simulink model "Our_model"  (R2024b)
settings: Solver=VariableStepAuto  StartTime=0.0  StopTime=50  MaxStep=0.01  RelTol=1e-3
model workspace: external: MATLAB File Non_Linear_Model_R2024a_saveas.m (data not in the file)
libraries: slpidlib x2
settings Model: Creator=tomkl  LastModifiedBy=tomkl

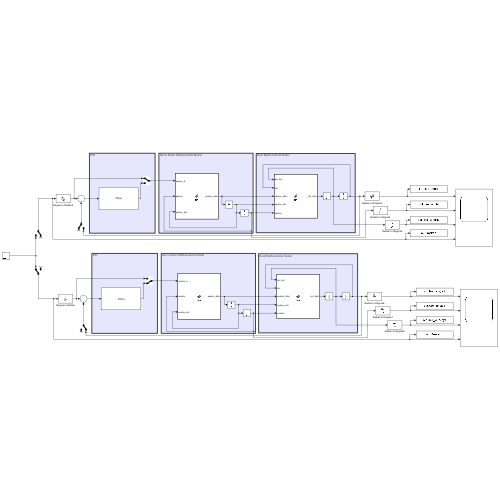
[thumbnail: Simulink's stored preview of the top-level diagram]
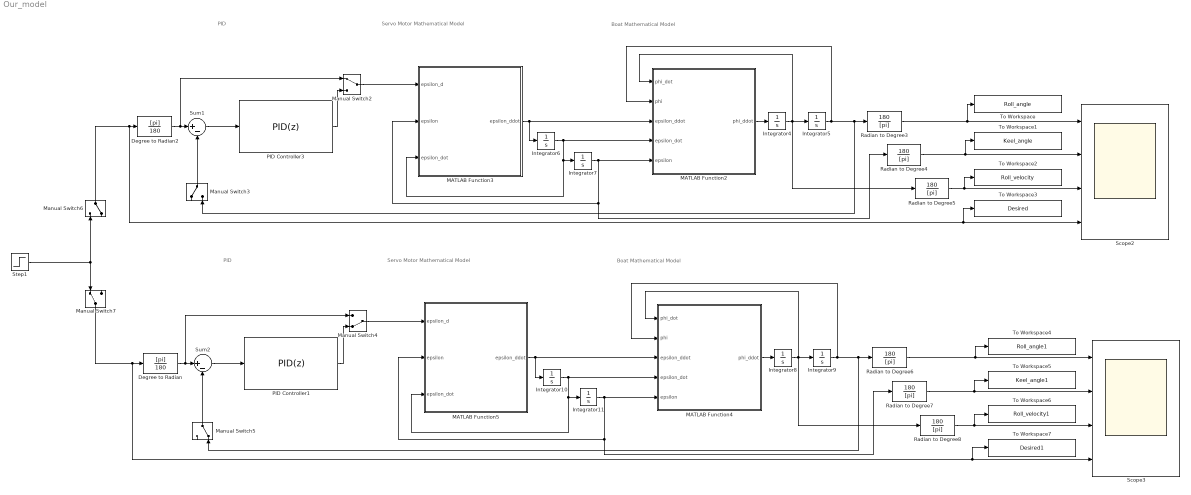
== system Our_model ==
  note: PID
  note: Boat Mathematical Model
  note: PID
  note: Servo Motor Mathematical Model
  note: Boat Mathematical Model
  note: Servo Motor Mathematical Model
  Degree to Radian : TransferFcn  Numerator=[pi]  Denominator=[180]
  Degree to Radian2 : TransferFcn  Numerator=[pi]  Denominator=[180]
  Integrator{4..11} (8 alike) : Integrator
  MATLAB Function2 : MATLAB Function  TreatAsAtomicUnit=on
  MATLAB Function3 : MATLAB Function  TreatAsAtomicUnit=on
  MATLAB Function4 : MATLAB Function  TreatAsAtomicUnit=on
  MATLAB Function5 : MATLAB Function  TreatAsAtomicUnit=on
  Manual Switch2 : ManualSwitch
  Manual Switch3 : ManualSwitch
  Manual Switch4 : ManualSwitch  CurrentSetting=0
  Manual Switch5 : ManualSwitch  CurrentSetting=0
  Manual Switch6 : ManualSwitch  CurrentSetting=0
  Manual Switch7 : ManualSwitch
  PID Controller1 : slpidlib/PID Controller  Controller=PID  Form=Parallel  TimeDomain=Discrete-time  UseExternalTs=off  SampleTime=0.01  IntegratorMethod=Forward Euler  FilterMethod=Forward Euler  ControllerParametersSource=internal  P=.8  I=0  UseKiTs=off  D=0  UseExternalDerivativeSource=off  N=1.7  UseFilter=on  TunerSelectOption=Transfer Function Based (PID Tuner App)  InitialConditionSource=internal  InitialConditionForIntegrator=0  InitialConditionForFilter=0  DifferentiatorICPrevScaledInput=0  ExternalReset=none  TrackingMode=off  Kt=1  LimitOutput=off  SatLimitsSource=internal  UpperSaturationLimit=inf  LowerSaturationLimit=-inf  LinearizeAsGain=on  AntiWindupMode=none  Kb=1  LimitIntegrator=off  UpperIntegratorSaturationLimit=inf  LowerIntegratorSaturationLimit=-inf  POutMin=[]  POutMax=[]  IOutMin=[]  IOutMax=[]  DOutMin=[]  DOutMax=[]  NOutMin=[]  NOutMax=[]  SumOutMin=[]  SumOutMax=[]  SaturationOutMin=[]  SaturationOutMax=[]  PParamMin=[]  PParamMax=[]  IParamMin=[]  IParamMax=[]  DParamMin=[]  DParamMax=[]  NParamMin=[]  NParamMax=[]  KbParamMin=[]  KbParamMax=[]  KtParamMin=[]  KtParamMax=[]  KbOutMin=[]  KbOutMax=[]  KtOutMin=[]  KtOutMax=[]  IntegratorOutMin=[]  IntegratorOutMax=[]  FilterOutMin=[]  FilterOutMax=[]  SumI1OutMin=[]  SumI1OutMax=[]  SumI2OutMin=[]  SumI2OutMax=[]  SumI3OutMin=[]  SumI3OutMax=[]  SumI4OutMin=[]  SumI4OutMax=[]  SumDOutMin=[]  SumDOutMax=[]  DifferentiatorOutMin=[]  DifferentiatorOutMax=[]  FilterDiffOutCoefMin=[]  FilterDiffOutCoefMax=[]  ReciprocalOutMin=[]  ReciprocalOutMax=[]  SumDenOutMin=[]  SumDenOutMax=[]  SumNumOutMin=[]  SumNumOutMax=[]  DivideOutMin=[]  DivideOutMax=[]  UdiffTsProdOutMin=[]  UdiffTsProdOutMax=[]  NTsProdOutMin=[]  NTsProdOutMax=[]  UintegralTsProdOutMin=[]  UintegralTsProdOutMax=[]  UngainTsProdOutMin=[]  UngainTsProdOutMax=[]  ClampingZeroOutDataTypeStr=Inherit: Inherit via back propagation  ClampingZeroOutMin=[]  ClampingZeroOutMax=[]  FilterDenConstantOutDataTypeStr=Inherit: Inherit via back propagation  FilterDenConstantOutMin=[]  FilterDenConstantOutMax=[]  PCopyOutDataTypeStr=Inherit: Inherit via back propagation  PCopyOutMin=[]  PCopyOutMax=[]  NCopyOutDataTypeStr=Inherit: Inherit via back propagation  NCopyOutMin=[]  NCopyOutMax=[]  IntegratorContinuousStateAttributes=''  IntegratorStateMustResolveToSignalObject=off  IntegratorRTWStateStorageClass=Auto  FilterContinuousStateAttributes=''  FilterStateMustResolveToSignalObject=off  FilterRTWStateStorageClass=Auto  ParallelPVariant=InternalParameters  IdealPVariant=Disabled  IVariant=InternalParameters  DVariant=InternalParameters  IntegratorVariant=Discrete  SatVariant=Disabled  AWVariant=Passthrough  PCopyVariant=Disabled  TRVariant=Disabled  FdbkBlocksVariant=Forward  IdealPFdbkVariant=Disabled  SatFdbkVariant=Disabled  DerivativeFilterVariant=ForwardEulerFilter  NVariant=InternalParameters  NCopyVariant=Disabled  FilterICVariant=InternalICsFilter  IntegratorICVariant=InternalICs  ExternalResetVariant=Disabled  TRSumVariant=Passthrough  SumFdbkVariant=Disabled  SumVariant=Sum_PID  TsampFilterVariant=InternalTs  TsampNgainVariant=Passthrough  TsampIntegralVariant=Disabled_SignalSpec  ExternalSaturationOutDataTypeStr=Inherit: Same as second input  DerivativeSourceVariant=ErrorSignal  PreIntVariant=InternalPreInt
  PID Controller3 : slpidlib/PID Controller  Controller=PID  Form=Parallel  TimeDomain=Discrete-time  UseExternalTs=off  SampleTime=0.01  IntegratorMethod=Forward Euler  FilterMethod=Forward Euler  ControllerParametersSource=internal  P=0.566467721992697  I=0.110964200934941  UseKiTs=off  D=0.339704255295508  UseExternalDerivativeSource=off  N=1.35164961739647  UseFilter=on  TunerSelectOption=Transfer Function Based (PID Tuner App)  InitialConditionSource=internal  InitialConditionForIntegrator=0  InitialConditionForFilter=0  DifferentiatorICPrevScaledInput=0  ExternalReset=none  TrackingMode=off  Kt=1  LimitOutput=off  SatLimitsSource=internal  UpperSaturationLimit=inf  LowerSaturationLimit=-inf  LinearizeAsGain=on  AntiWindupMode=none  Kb=1  LimitIntegrator=off  UpperIntegratorSaturationLimit=inf  LowerIntegratorSaturationLimit=-inf  POutMin=[]  POutMax=[]  IOutMin=[]  IOutMax=[]  DOutMin=[]  DOutMax=[]  NOutMin=[]  NOutMax=[]  SumOutMin=[]  SumOutMax=[]  SaturationOutMin=[]  SaturationOutMax=[]  PParamMin=[]  PParamMax=[]  IParamMin=[]  IParamMax=[]  DParamMin=[]  DParamMax=[]  NParamMin=[]  NParamMax=[]  KbParamMin=[]  KbParamMax=[]  KtParamMin=[]  KtParamMax=[]  KbOutMin=[]  KbOutMax=[]  KtOutMin=[]  KtOutMax=[]  IntegratorOutMin=[]  IntegratorOutMax=[]  FilterOutMin=[]  FilterOutMax=[]  SumI1OutMin=[]  SumI1OutMax=[]  SumI2OutMin=[]  SumI2OutMax=[]  SumI3OutMin=[]  SumI3OutMax=[]  SumI4OutMin=[]  SumI4OutMax=[]  SumDOutMin=[]  SumDOutMax=[]  DifferentiatorOutMin=[]  DifferentiatorOutMax=[]  FilterDiffOutCoefMin=[]  FilterDiffOutCoefMax=[]  ReciprocalOutMin=[]  ReciprocalOutMax=[]  SumDenOutMin=[]  SumDenOutMax=[]  SumNumOutMin=[]  SumNumOutMax=[]  DivideOutMin=[]  DivideOutMax=[]  UdiffTsProdOutMin=[]  UdiffTsProdOutMax=[]  NTsProdOutMin=[]  NTsProdOutMax=[]  UintegralTsProdOutMin=[]  UintegralTsProdOutMax=[]  UngainTsProdOutMin=[]  UngainTsProdOutMax=[]  ClampingZeroOutDataTypeStr=Inherit: Inherit via back propagation  ClampingZeroOutMin=[]  ClampingZeroOutMax=[]  FilterDenConstantOutDataTypeStr=Inherit: Inherit via back propagation  FilterDenConstantOutMin=[]  FilterDenConstantOutMax=[]  PCopyOutDataTypeStr=Inherit: Inherit via back propagation  PCopyOutMin=[]  PCopyOutMax=[]  NCopyOutDataTypeStr=Inherit: Inherit via back propagation  NCopyOutMin=[]  NCopyOutMax=[]  IntegratorContinuousStateAttributes=''  IntegratorStateMustResolveToSignalObject=off  IntegratorRTWStateStorageClass=Auto  FilterContinuousStateAttributes=''  FilterStateMustResolveToSignalObject=off  FilterRTWStateStorageClass=Auto  ParallelPVariant=InternalParameters  IdealPVariant=Disabled  IVariant=InternalParameters  DVariant=InternalParameters  IntegratorVariant=Discrete  SatVariant=Disabled  AWVariant=Passthrough  PCopyVariant=Disabled  TRVariant=Disabled  FdbkBlocksVariant=Forward  IdealPFdbkVariant=Disabled  SatFdbkVariant=Disabled  DerivativeFilterVariant=ForwardEulerFilter  NVariant=InternalParameters  NCopyVariant=Disabled  FilterICVariant=InternalICsFilter  IntegratorICVariant=InternalICs  ExternalResetVariant=Disabled  TRSumVariant=Passthrough  SumFdbkVariant=Disabled  SumVariant=Sum_PID  TsampFilterVariant=InternalTs  TsampNgainVariant=Passthrough  TsampIntegralVariant=Disabled_SignalSpec  ExternalSaturationOutDataTypeStr=Inherit: Same as second input  DerivativeSourceVariant=ErrorSignal  PreIntVariant=InternalPreInt
  Radian to Degree{3..8} (6 alike) : TransferFcn  Numerator=[180]  Denominator=[pi]
  Scope2 : Scope  NumInputPorts=4
  Scope3 : Scope  NumInputPorts=4
  Step1 : Step  SampleTime=0
  Sum1 : Sum  Inputs=|+-
  Sum2 : Sum  Inputs=|+-
  To Workspace : ToWorkspace  VariableName=Roll_angle  SaveFormat=Timeseries  SampleTime=-1
  To Workspace1 : ToWorkspace  VariableName=Keel_angle  SaveFormat=Timeseries  SampleTime=-1
  To Workspace2 : ToWorkspace  VariableName=Roll_velocity  SaveFormat=Timeseries  SampleTime=-1
  To Workspace3 : ToWorkspace  VariableName=Desired  SaveFormat=Timeseries  SampleTime=-1
  To Workspace4 : ToWorkspace  VariableName=Roll_angle1  SaveFormat=Timeseries  SampleTime=-1
  To Workspace5 : ToWorkspace  VariableName=Keel_angle1  SaveFormat=Timeseries  SampleTime=-1
  To Workspace6 : ToWorkspace  VariableName=Roll_velocity1  SaveFormat=Timeseries  SampleTime=-1
  To Workspace7 : ToWorkspace  VariableName=Desired1  SaveFormat=Timeseries  SampleTime=-1
  wires:
  Sum1/1 -> PID Controller3/1
  Integrator11/1 -> Radian to Degree7/1, MATLAB Function5/2(epsilon), MATLAB Function4/5(epsilon)
  Radian to Degree5/1 -> Scope2/3, To Workspace2/1
  Integrator8/1 -> Radian to Degree8/1, MATLAB Function4/1(phi_dot), Integrator9/1
  Radian to Degree4/1 -> To Workspace1/1, Scope2/2
  MATLAB Function3/1(epsilon_ddot) -> Integrator6/1, MATLAB Function2/3(epsilon_ddot)
  Manual Switch4/1 -> MATLAB Function5/1(epsilon_d)
  Manual Switch5/1 -> Sum2/2
  Manual Switch7/1 -> Scope3/4, To Workspace7/1, Degree to Radian/1
  Integrator4/1 -> Radian to Degree5/1, MATLAB Function2/1(phi_dot), Integrator5/1
  MATLAB Function2/1(phi_ddot) -> Integrator4/1
  Radian to Degree7/1 -> Scope3/2, To Workspace5/1
  Sum2/1 -> PID Controller1/1
  Degree to Radian2/1 -> Manual Switch2/1, Sum1/1
  Integrator9/1 -> Radian to Degree6/1, Manual Switch5/2, MATLAB Function4/2(phi)
  PID Controller3/1 -> Manual Switch2/2
  Manual Switch3/1 -> Sum1/2
  Manual Switch2/1 -> MATLAB Function3/1(epsilon_d)
  Integrator6/1 -> MATLAB Function2/4(epsilon_dot), MATLAB Function3/3(epsilon_dot), Integrator7/1
  Integrator10/1 -> MATLAB Function4/4(epsilon_dot), MATLAB Function5/3(epsilon_dot), Integrator11/1
  Integrator7/1 -> Radian to Degree4/1, MATLAB Function3/2(epsilon), MATLAB Function2/5(epsilon)
  MATLAB Function5/1(epsilon_ddot) -> Integrator10/1, MATLAB Function4/3(epsilon_ddot)
  Step1/1 -> Manual Switch6/1, Manual Switch7/1
  Degree to Radian/1 -> Manual Switch4/1, Sum2/1
  Radian to Degree3/1 -> Scope2/1, To Workspace/1
  Radian to Degree8/1 -> Scope3/3, To Workspace6/1
  Manual Switch6/1 -> Scope2/4, To Workspace3/1, Degree to Radian2/1
  MATLAB Function4/1(phi_ddot) -> Integrator8/1
  Radian to Degree6/1 -> To Workspace4/1, Scope3/1
  PID Controller1/1 -> Manual Switch4/2
  Integrator5/1 -> Manual Switch3/2, Radian to Degree3/1, MATLAB Function2/2(phi)

== matlab function Our_model/MATLAB Function2 ==
  data: phi_dot input; phi input; epsilon_ddot input; epsilon_dot input; phi_ddot output; epsilon input
function phi_ddot=fcn(phi_dot, phi, epsilon_ddot, epsilon_dot, epsilon)

%defining contants
rhi = 1025;           %Density of sea water [kg/m^3]
g = 9.81;             %Gravity [m/s^2]

I_x = 0.0005589;      %Roll moment of inertia of the vessel [kgm^2]         %from Juan
delta_I_x = 0.0001567;%Hydrodynamic added mass coefficient  [kgm^2]         %from Juan
nabla = 1.150/rhi;    %Volume displacement of the ship [kg]                 %from Juan
GMm_bar = 0.2251;     %Mean metacentric height [m]                          %from Juan
K_dphi = 0.568;       %Linear positive drag coefficient in roll [kgm^2/s]   %from Juan
K_dphidphi = 0.284;   %Non-linear positive drag coefficient in roll [kgm^2] %from Juan  

m_k = 0.0803;         %Mass of the keel system [kg]
nabla_k = 0.0003;     %Volume of the keel system [m^3]
z_k = 0.06;           %Distance between the vessels center of mass and the hinge point of the keel [m]                 
L_k = 0.215;          %Distance between the hinge point to the mass/buoancy center of keel system [m]

J_km = 0.00002;       %Motor intertia coefficient [kgm^2]
B_km = 0.10;           %Motor damping coefficient [NMs/rad]

m_d = 0.1;            %Mass of the load in the vessel frame [kgs]
y_d = 0.07;           %Lateral position of the load of mass in the vessel frame [m]
z_d = 0.0472;         %Vertical position of the load of mass from the center of mass of the vessel [m]
    

K_phi3 = 3;             %Not specified                                      %from paper which they guessed 
K_k = 0.05;            %Linear drag coefficient                            %scaled down from paper
K_kk = 0.025;          %Non linear drag coefficient                        %scaled down from paper

delta_m_k = nabla*rhi;

%defining function
phi_ddot = ( ...
    -K_dphi*phi_dot ...
    -K_dphidphi*phi_dot*abs(phi_dot) ...
    -rhi*g*nabla*GMm_bar*phi ...
    -K_phi3*phi^3 ...
    -(m_k-rhi*nabla_k)*g*(z_k*sin(phi)+L_k*sin(epsilon+phi)) ...
    -K_k*(epsilon_dot+phi_dot) -K_kk*(epsilon_dot+phi_dot)*abs(epsilon_dot-phi_dot) ...
    -J_km*epsilon_ddot-B_km*epsilon_dot ...
    +0*m_d*g*(z_d*sin(phi)+y_d*cos(phi)) ...
    -delta_m_k*epsilon_ddot)/(I_x+delta_I_x+delta_m_k);

== matlab function Our_model/MATLAB Function3 ==
  data: epsilon_d input; epsilon input; epsilon_dot input; epsilon_ddot output
function epsilon_ddot=fcn(epsilon_d,epsilon,epsilon_dot)

%defining contants
u=epsilon_d;                       %input value
k_t = 0.065;                       %Motor torque constant [Nm/A]          %calculated from datasheet
k_pm = 1000;                          %Motor controller proportional gain    %from paper
J_km = 0.00002;                    %Motor inertia coefficient [kgm^2]     %from Juan data
R_a = 2.61;                        %Motor armature resistance [ohm]       %chatgpt calculations
k_b = 1.02;                        %Motor Back-Emf constant [Vs/rad]      %chatgpt estimated 
k_dm = 0.5;                        %Motor controller derivative gain      %from paper
B_km = 0.10;                        %Motor damping coefficient [Nms/rad]   %from Juan


alpha_1 = (-k_t*k_pm)/(J_km*R_a);
alpha_2 = (-k_t*(k_b+k_dm)-R_a*B_km)/(J_km*R_a);
Beta = (k_t*k_pm)/(J_km*R_a);

%J_km, B_km are in both function block, care for it while changing values

%defining funciton
epsilon_ddot=alpha_1*epsilon+alpha_2*epsilon_dot+Beta*u;

== matlab function Our_model/MATLAB Function4 ==
  data: phi_dot input; phi input; epsilon_ddot input; epsilon_dot input; phi_ddot output; epsilon input
function phi_ddot=fcn(phi_dot, phi, epsilon_ddot, epsilon_dot, epsilon)

%defining contants
rhi = 1025;           %Density of sea water [kg/m^3]
g = 9.81;             %Gravity [m/s^2]

I_x = 0.0005589;      %Roll moment of inertia of the vessel [kgm^2]         %from Juan
delta_I_x = 0.0001567;%Hydrodynamic added mass coefficient  [kgm^2]         %from Juan
nabla = 1.150/rhi;    %Volume displacement of the ship [kg]                 %from Juan
GMm_bar = 0.2251;     %Mean metacentric height [m]                          %from Juan
K_dphi = 0.568;       %Linear positive drag coefficient in roll [kgm^2/s]   %from Juan
K_dphidphi = 0.284;   %Non-linear positive drag coefficient in roll [kgm^2] %from Juan  

m_k = 0.0803;         %Mass of the keel system [kg]
nabla_k = 0.0003;     %Volume of the keel system [m^3]
z_k = 0.06;           %Distance between the vessels center of mass and the hinge point of the keel [m]                 
L_k = 0.215;          %Distance between the hinge point to the mass/buoancy center of keel system [m]

J_km = 0.00002;       %Motor intertia coefficient [kgm^2]
B_km = 0.10;           %Motor damping coefficient [NMs/rad]

m_d = 0.1;            %Mass of the load in the vessel frame [kgs]
y_d = 0.07;           %Lateral position of the load of mass in the vessel frame [m]
z_d = 0.0472;         %Vertical position of the load of mass from the center of mass of the vessel [m]
    

K_phi3 = 3;             %Not specified                                      %from paper which they guessed 
K_k = 0.05;            %Linear drag coefficient                            %scaled down from paper
K_kk = 0.025;          %Non linear drag coefficient                        %scaled down from paper

delta_m_k = nabla*rhi;

%defining function
phi_ddot = ( ...
    -K_dphi*phi_dot ... 
    -rhi*g*nabla*GMm_bar*phi ...
    -(m_k-rhi*nabla_k)*g*(z_k*(phi)+L_k*(epsilon+phi)) ...
    -K_k*(epsilon_dot+phi_dot)...
    -J_km*epsilon_ddot-B_km*epsilon_dot ...
    -delta_m_k*epsilon_ddot)/(I_x+delta_I_x+delta_m_k);

== matlab function Our_model/MATLAB Function5 ==
  data: epsilon_d input; epsilon input; epsilon_dot input; epsilon_ddot output
function epsilon_ddot=fcn(epsilon_d,epsilon,epsilon_dot)

%defining variables
u=epsilon_d;                       %input value
k_t = 0.65;                       %Motor torque constant [Nm/A]          %calculated from datasheet
k_pm = 1000;                          %Motor controller proportional gain    %from paper
J_km = 0.00002;                    %Motor inertia coefficient [kgm^2]     %from Juan data
R_a = 2.61;                        %Motor armature resistance [ohm]       %chatgpt calculations
k_b = 1.02;                        %Motor Back-Emf constant [Vs/rad]      %chatgpt estimated 
k_dm = 0.3;                        %Motor controller derivative gain      %from paper
B_km = 0.10;                        %Motor damping coefficient [Nms/rad]   %from Juan

alpha_1 = (-k_t*k_pm)/(J_km*R_a);
alpha_2 = (-k_t*(k_b+k_dm)-R_a*B_km)/(J_km*R_a);
Beta = (k_t*k_pm)/(J_km*R_a);

%J_km, B_km are in both function block, care for it while changing values

%defining funciton
epsilon_ddot=alpha_1*epsilon+alpha_2*epsilon_dot+Beta*u;
